simulink model "Z_3Dctrl"  (R2023a)
settings: Solver=ode1  StartTime=0.0  StopTime=inf  FixedStep=0.001  RelTol=1e-3  EnableMultiTasking=on
PostLoadFcn:
  | , if any(exist('dsrtsu_mdlpostloadfcn', 'file') ~= 0), dsrtsu_mdlpostloadfcn('Execute', bdroot); end,
InitFcn:
  | , if any(exist('rtifpga_mdlclblib', 'file') ~= 0), rtifpga_mdlclblib('Init', bdroot); end,
  | [b,a] = butter(6,0.6)
  | z0_default = 0.080001
  | fatness_default = 1
  | offset_default = 0
  | scale_default = 0
  | tic
model workspace (MAT data in the model file):
  Iters = 5
  N_coils = 6
  fatness_default = 1
  running = 0
  z0_default = 0.080001
undefined symbols (not defined in the file or in its folder): a, b, DiscIntNeverNeededParam
libraries: dspstat3 x7, simulink x5, commfilt2 x3, rti2004lib x3, rtilibm x1
(part 1 of 3)
settings Model: DSRTSU_INTERNAL_RTI_VER=620  DSRTSU_INTERNAL_RTI_TYPE=rti1006  DSRTSU_INTERNAL_RTIFPGA=200  DSRTSU_INTERNAL_RTISTBM_VER=23.1  Creator=Administrator  LastModifiedBy=inst
settings SolverCC: AlgebraicLoopSolver=TrustRegion
settings DataIOCC: LimitDataPoints=on  SaveFormat=Array  SignalLoggingSaveFormat=ModelDataLogs  ReturnWorkspaceOutputs=off
settings OptimizationCC: BlockReduction=off  OptimizeBlockIOStorage=off  BufferReuse=off  ReuseModelBlockBuffer=off  ExpressionFolding=off  ExpressionDepthLimit=2147483647  LocalBlockOutputs=off  LifeSpan=inf
settings DebuggingCC: UnderspecifiedInitializationDetection=Classic  MergeDetectMultiDrivingBlocksExec=none  SolverPrmCheckMsg=warning  FcnCallInpInsideContextMsg=warning  UnconnectedInputMsg=warning  UnconnectedOutputMsg=warning  UnconnectedLineMsg=warning  StateNameClashWarn=warning  SFUnexpectedBacktrackingDiag=warning  SFNoUnconditionalDefaultTransitionDiag=warning  SFExecutionAtInitializationDiag=none  ArithmeticOperatorsInVariantConditions=warning
settings HardwareCC: ProdBitPerPointer=32  ProdBitPerSizeT=32  ProdBitPerPtrDiffT=32  ProdLargestAtomicInteger=Integer  ProdWordSize=32  ProdHWDeviceType=Custom Processor->Custom  TargetIntDivRoundTo=Zero  TargetEndianess=LittleEndian  TargetHWDeviceType=Custom Processor->Custom
settings ModelReferenceCC: EnableRefExpFcnMdlSchedulingChecks=on  PropagateSignalLabelsOutOfModel=off
settings SFSimCC: SimUseLocalCustomCode=off  MATLABDynamicMemAlloc=off  CustomCodeUndefinedFunction=UseInterfaceOnly
settings RTWCC: Description=dSPACE DS1006 Hardware Platform  SystemTargetFile=rti1006.tlc  MakeCommand=make_rti  TemplateMakefile=rti1006.tmf  RTWUseLocalCustomCode=off
settings CodeAppCC: StateflowObjectComments=on
settings STFCustomTargetCC: TargetLangStandard=C89/C90 (ANSI)  ParMdlRefBuildCompliant=on  ConcurrentExecutionCompliant=off  GRTInterface=off  UseToolchainInfoCompliant=off  SystemTargetFile=rti1006.tlc
settings GRTTargetCC: TargetLangStandard=C89/C90 (ANSI)  CompOptLevelCompliant=off  ConcurrentExecutionCompliant=off  CombineOutputUpdateFcns=off  MatFileLogging=off  CPPClassGenCompliant=off  UseToolchainInfoCompliant=off  ExtModeMexFile=noextcomm
settings ConfigComp: CovMetricSettings=dw  CovSaveCumulativeToWorkspaceVar=on  CovSaveSingleToWorkspaceVar=on

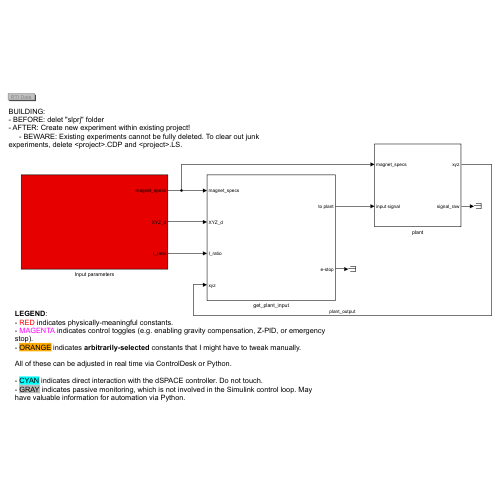
[thumbnail: Simulink's stored preview of the top-level diagram]
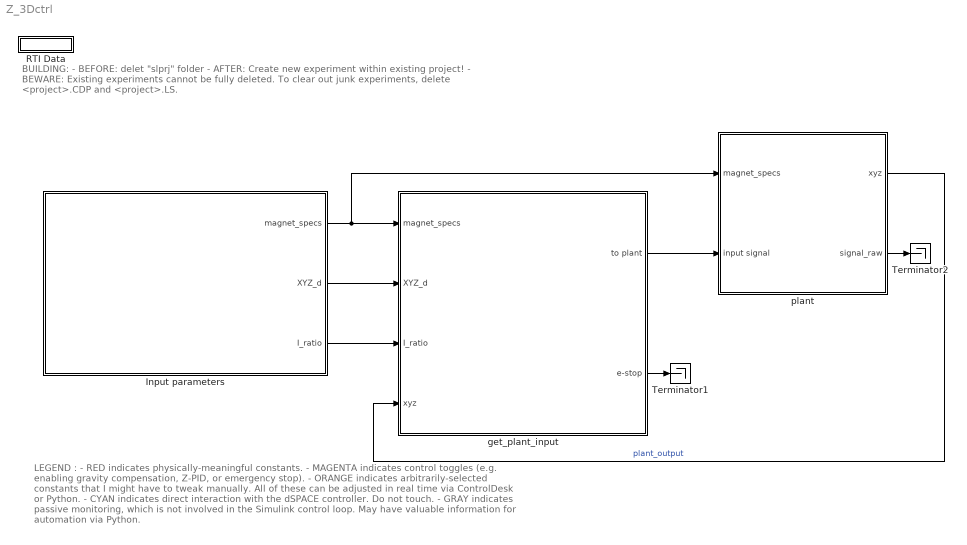
== system Z_3Dctrl ==
  note: BUILDING:
      | - BEFORE: delet "slprj" folder
      | - AFTER: Create new experiment within existing project!
      | - BEWARE: Existing experiments cannot be fully deleted. To clear out junk experiments, delete <project>.CDP and <project>.LS.
  note: LEGEND :
      | - RED indicates physically-meaningful constants.
      | - MAGENTA indicates control toggles (e.g. enabling gravity compensation, Z-PID, or emergency stop).
      | - ORANGE indicates arbitrarily-selected constants that I might have to tweak manually.
      |
      | All of these can be adjusted in real time via ControlDesk or Python.
      |
      | - CYAN indicates direct interaction with the dSPACE controller. Do not touch.
      | - GRAY indicates passive monitoring, which is not involved in the Simulink control loop. May have valuable information for automation via Python.
  Input parameters : Subsystem
  RTI Data : Subsystem  Tag=struct('RTIDataServer',struct('RTIDataServerVs','2','RTIModelDescription','struct(''main'',''Z_1Dctrl_simplified'',''sub'','''',''isMp'',0)'))  LoadFcn="if exist('rtidc'), try,  rtidc('DataHostBlockClbLoad', gcbh); catch, disp(['Warning: ''LoadFcn'' for RTI Data block failed: ' lasterr]); end, end,"  mask(RTI_DATA_HOST){}
      mask help:
      | RTI Data Block.
      | This block is used by RTI to store internal model-dependent data.
      | Please keep this block on the root level of the model. Deleting this block will result in data loss.
      |
      | NEVER DELETE OR COPY THIS BLOCK!
      settings: CopyFcn="if exist('rtidc'), try,  rtidc('DataHostBlockClbCopy', gcbh); catch, disp(['Warning: ''CopyFcn'' for RTI Data block failed: ' lasterr]); end, end,"  DeleteFcn="if exist('rtidc'), try,  rtidc('DataHostBlockClbDelete', gcbh); catch, disp(['Warning: ''DeleteFcn'' for RTI Data block failed: ' lasterr]); end, end,"  ModelCloseFcn="if exist('rtidc'), try,  rtidc('DataHostBlockClbModelClose', gcbh); catch, disp(['Warning: ''ModelCloseFcn'' for RTI Data block failed: ' lasterr]); end, end,"  PreSaveFcn="if exist('rtidc'), try,  rtidc('DataHostBlockClbPreSave', gcbh); catch, disp(['Warning: ''PreSaveFcn'' for RTI Data block failed: ' lasterr]); end, end,"  PostSaveFcn="if exist('rtidc'), try,  rtidc('DataHostBlockClbPostSave', gcbh); catch, disp(['Warning: ''PostSaveFcn'' for RTI Data block failed: ' lasterr]); end, end,"  NameChangeFcn="if exist('rtidc'), try,  rtidc('DataHostBlockClbNameChange', gcbh); catch, disp(['Warning: ''NameChangeFcn'' for RTI Data block failed: ' lasterr]); end, end,"
      mask Help:
      | RTI Data Block.
      | This block is used by RTI to store internal model-dependent data.
      | Please keep this block on the root level of the model. Deleting this block will result in data loss.
      | 
      | NEVER DELETE OR COPY THIS BLOCK!
      mask Display:
      | text(0.5, 0.5, 'RTI Data', 'HorizontalAlignment', 'center');
      | plot([1 0]);
  Terminator1 : Terminator
  Terminator2 : Terminator
  get_plant_input : Subsystem
  plant : Subsystem
  wires:
  Input parameters/1(magnet_specs) -> plant/1(magnet_specs), get_plant_input/1(magnet_specs)
  Input parameters/2(XYZ_d) -> get_plant_input/2(XYZ_d)
  plant/1(xyz) -> get_plant_input/4(xyz)  "plant_output"
  Input parameters/3(I_ratio) -> get_plant_input/3(I_ratio)
  get_plant_input/1(to plant) -> plant/2(input signal)
  get_plant_input/2(e-stop) -> Terminator1/1
  plant/2(signal_raw) -> Terminator2/1

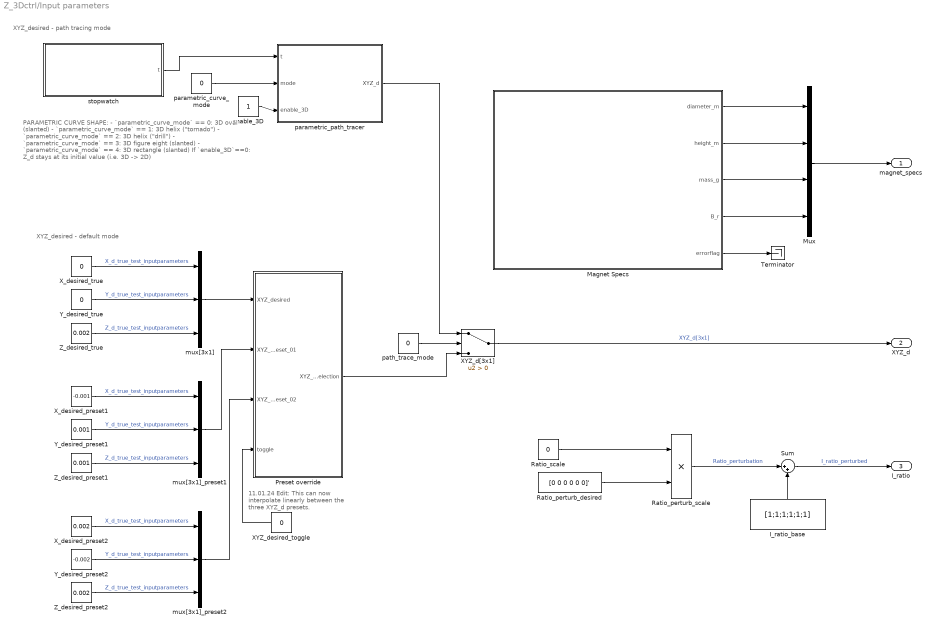
== system Z_3Dctrl/Input parameters ==
  note: XYZ_desired - path tracing mode
  note: PARAMETRIC CURVE SHAPE:
      | - `parametric_curve_mode` == 0: 3D oval (slanted)
      | - `parametric_curve_mode` == 1: 3D helix ("tornado")
      | - `parametric_curve_mode` == 2: 3D helix ("drill")
      | - `parametric_curve_mode` == 3: 3D figure eight (slanted)
      | - `parametric_curve_mode` == 4: 3D rectangle (slanted)
      |
      | If `enable_3D`==0: Z_d stays at its initial value (i.e. 3D -> 2D)
  note: XYZ_desired - default mode
  note: 11.01.24 Edit:
      | This can now interpolate linearly between the three XYZ_d presets.
  I_ratio_base : Constant  Value=[1;1;1;1;1;1]
  Magnet Specs : Subsystem
  Mux : Mux
  Preset override : MATLAB Function  TreatAsAtomicUnit=on
  Ratio_perturb_desired : Constant  Value=[0 0 0 0 0 0]'
  Ratio_perturb_scale : Product
  Ratio_scale : Constant  Value=0
  Sum : Sum  Inputs=|++
  Terminator : Terminator
  XYZ_d[3x1] : Switch  Criteria=u2 > Threshold  SaturateOnIntegerOverflow=off  InputSameDT=off
  XYZ_desired_toggle : Constant  Value=0
  X_desired_preset1 : Constant  Value=-0.001
  X_desired_preset2 : Constant  Value=0.002
  X_desired_true : Constant  Value=0
  Y_desired_preset1 : Constant  Value=0.001
  Y_desired_preset2 : Constant  Value=-0.002
  Y_desired_true : Constant  Value=0
  Z_desired_preset1 : Constant  Value=0.001
  Z_desired_preset2 : Constant  Value=0.002
  Z_desired_true : Constant  Value=0.002
  enable_3D : Constant
  mux[3x1] : Mux  Inputs=3
  mux[3x1]_preset1 : Mux  Inputs=3
  mux[3x1]_preset2 : Mux  Inputs=3
  parametric_curve_mode : Constant  Value=0
  parametric_path_tracer : MATLAB Function  TreatAsAtomicUnit=on
  path_trace_mode : Constant  Value=0
  stopwatch : Subsystem
  magnet_specs : Outport
  XYZ_d : Outport  Port=2
  I_ratio : Outport  Port=3
  wires:
  Magnet Specs/1(diameter_m) -> Mux/1
  Magnet Specs/2(height_m) -> Mux/2
  Magnet Specs/3(mass_g) -> Mux/3
  Magnet Specs/4(B_r) -> Mux/4
  Mux/1 -> magnet_specs/1
  Magnet Specs/5(errorflag) -> Terminator/1
  Z_desired_true/1 -> mux[3x1]/3  "Z_d_true_test_inputparameters"
  Ratio_scale/1 -> Ratio_perturb_scale/1
  Ratio_perturb_desired/1 -> Ratio_perturb_scale/2
  Sum/1 -> I_ratio/1  "I_ratio_perturbed"
  I_ratio_base/1 -> Sum/2
  Ratio_perturb_scale/1 -> Sum/1  "Ratio_perturbation"
  Y_desired_true/1 -> mux[3x1]/2  "Y_d_true_test_inputparameters"
  X_desired_true/1 -> mux[3x1]/1  "X_d_true_test_inputparameters"
  mux[3x1]/1 -> Preset override/1(XYZ_desired)
  Preset override/1(XYZ_desired_selection) -> XYZ_d[3x1]/3
  X_desired_preset1/1 -> mux[3x1]_preset1/1  "X_d_true_test_inputparameters"
  Y_desired_preset1/1 -> mux[3x1]_preset1/2  "Y_d_true_test_inputparameters"
  mux[3x1]_preset1/1 -> Preset override/2(XYZ_preset_01)
  Z_desired_preset1/1 -> mux[3x1]_preset1/3  "Z_d_true_test_inputparameters"
  mux[3x1]_preset2/1 -> Preset override/3(XYZ_preset_02)
  Y_desired_preset2/1 -> mux[3x1]_preset2/2  "Y_d_true_test_inputparameters"
  X_desired_preset2/1 -> mux[3x1]_preset2/1  "X_d_true_test_inputparameters"
  Z_desired_preset2/1 -> mux[3x1]_preset2/3  "Z_d_true_test_inputparameters"
  XYZ_desired_toggle/1 -> Preset override/4(toggle)
  XYZ_d[3x1]/1 -> XYZ_d/1  "XYZ_d[3x1]"
  path_trace_mode/1 -> XYZ_d[3x1]/2
  stopwatch/1(t) -> parametric_path_tracer/1(t)
  parametric_curve_mode/1 -> parametric_path_tracer/2(mode)
  enable_3D/1 -> parametric_path_tracer/3(enable_3D)
  parametric_path_tracer/1(XYZ_d) -> XYZ_d[3x1]/1

== system Z_3Dctrl/RTI Data ==
  RTI Data Store : Subsystem  Tag="struct('private',struct('version',struct('dsVer',uint32(2),'dsVerCreation',uint32(2),'RTI',struct('ver','6.2','type','RTI1006')),'access',struct('type','Model','isPerm',1,'created',['29-Jul-2010 10:53:51'],'modified',['20-Nov-2024 19:16:55'],'location','')),'public',struct('main',struct('data',[]),'sub',struct('name',{{'Z_1Dctrl_simplified'}},'data',{{struct('TH',struct('thTaskInfo',struct('taskType',{'TIMER','HWINT','TMRINT','SWINT','GLINT'},'tasksNumOf',{1,0,0,0,0},'srcIds',{{'TIMERA'},{},{},{},{}},'taskNames',{{['Timer Task 1']},{},{},{},{}})),'th_tc',struct('dataType','TASK','taskGroupId','','taskGroupList',{{}},'taskSchedulingPolicy','FCFS','taskType','TIMER','blkh',-1,'srcId','TIMERA','srcSgnName',['Timer A interrupt'],'srcCpuName','','taskName',['Timer Task 1  [0.001] s'],'taskNameDisplayExt','','smplTime',0.001,'smplTimeOffs',0,'hasFixedPriority',0,'priority',1,'hasFixedOvc',0,'ovcType',1,'ovcMax',1),'tc_th',struct('dataType','TASK','taskGroupId','','taskGroupList',{{}},'taskSchedulingPolicy','FCFS','taskType','TIMER','blkh',-1,'srcId','TIMERA','srcSgnName',['Timer A interrupt'],'srcCpuName','','taskName',['Timer Task 1  [0.001] s'],'taskNameDisplayExt','','smplTime',0.001,'smplTimeOffs',0,'hasFixedPriority',0,'priority',1,'hasFixedOvc',0,'ovcType',1,'ovcMax',1))}})))"  mask(RTI_DATA_STORE){}
      mask help:
      | RTI Data Store Block. This block is used by RTI to store internal model dependent data. Deleting this block will result in data loss.
      |
      | NEVER DELETE, COPY, OR MODIFY THIS BLOCK!
      mask Help:
      | RTI Data Store Block. This block is used by RTI to store internal model dependent data. Deleting this block will result in data loss.
      | 
      | NEVER DELETE, COPY, OR MODIFY THIS BLOCK!
      mask Display: text(0.5, 0.5, ' ', 'HorizontalAlignment', 'center');

== system Z_3Dctrl/get_plant_input ==
  note: Inputs
  magnet_specs : Inport
  XYZ_d : Inport  Port=2
  I_ratio : Inport  Port=3
  xyz : Inport  Port=4
  Z_1dctrl : Subsystem
  to plant : Outport
  e-stop : Outport  Port=2
  wires:
  XYZ_d/1 -> Z_1dctrl/4(XYZd)
  xyz/1 -> Z_1dctrl/3(xyz)
  Z_1dctrl/1(to plant) -> to plant/1
  magnet_specs/1 -> Z_1dctrl/1(magnet specs)
  I_ratio/1 -> Z_1dctrl/2(I_ratio)
  Z_1dctrl/2(e-stop) -> e-stop/1

== system Z_3Dctrl/plant ==
  note: NOTE:
      | Output signal contains:
      | - x_pos : Centered, smoothed "x" [m] (not used in control yet)
      | - y_pos : Centered, smoothed "y" [m] (not used in control yet)
      | - z_pos : Centered, smoothed "z" [m] (to be used in derivative-related calculations ONLY)
      | - z_pos_raw : Centered but otherwise unprocessed "z" [m] (to be used in "PI" ONLY)
  magnet_specs : Inport  PortDimensions=[1 4]
  input signal : Inport  Port=2
  DS2103_B1 : rtilibm/DS2103/DS2103_B1  BoardNo=1  ChannelNos=[1 2 4 6 8 9 10 11 12 18 19 20]  Range=[10 10 10 10 10 10 10 10 10 10 10 10 10 10 10 10 10 10 10 10 10 10 10 10 10 10 10 10 10 10 10 10]  IOErrorMode=[1 1 1 1 1 1 1 1]  InitValue=[0 0 0 0 0 0 0 0 0 0 0 0 0 0 0 0 0 0 0 0 0 0 0 0 0 0 0 0 0 0 0 0]  TermMode=[0 0 0 0 0 0 0 1 1 1 1 1 1 1 1 1 1 1 1 1 1 1 1 1 1 1 1 1 1 1 1 1]  TermValue=[0 0 0 0 0 0 0 0 0 0 0 0 0 0 0 0 0 0 0 0 0 0 0 0 0 0 0 0 0 0 0 0]  DialogFcn=gui2103  UnitName={ 'DS2103_B' }  UnitValues={ 1 }  DSProperties=struct('RTI',struct('Version',uint32(1),'BlockType',struct('isSLSource',uint8(0),'isSLSink',uint8(1),'isHWSource',uint8(0),'isHWSink',uint8(1),'isSetup',uint8(0),'isInline',uint8(1),'isNonInline',uint8(0),'isInterrupt',uint8(0),'isChannelwise',uint8(0)),'IOBoardType','DS2103','UnitType','DAC','Identifier','DACMUX','DialogType','ML','BlockSet','NONE','SlaveProcessor','NONE'))
      settings: SourceProductName=dSPACE RTI1006
  Demux : Demux
  Mux : Mux  Inputs=3
  Position Determination1 : Subsystem  TreatAsAtomicUnit=on
  Terminator : Terminator
  Terminator2 : Terminator
  output signal : Subsystem
  xyz : Outport
  signal_raw : Outport  Port=2
  wires:
  input signal/1 -> DS2103_B1/1
  Demux/4 -> Terminator/1  "B_r"
  Demux/1 -> Position Determination1/1(height_m)  "diameter_m"
  Demux/2 -> Position Determination1/2(diameter_m)  "height_m"
  Demux/3 -> Terminator2/1  "mass_g"
  Position Determination1/1(x_SAR(m)) -> Mux/1  "x_SAR"
  Position Determination1/2(y_SAR(m)) -> Mux/2  "y_SAR"
  Position Determination1/3(z_SAR(m)) -> Mux/3  "z_SAR"
  output signal/1(plant signals) -> signal_raw/1, Position Determination1/3(plant signals)
  Mux/1 -> xyz/1
  magnet_specs/1 -> Demux/1

== system Z_3Dctrl/Input parameters/Magnet Specs ==
  note: NOTE: Xiaodong lists the magnet as having 10mm height and 10mm diameter. However, height is closer to 11-12mm. Diameter is closer to ????.
  Diameter : Constant  Value=0.635
  Height : Constant  Value=0.635
  Magnet Physical Specs : MATLAB Function  TreatAsAtomicUnit=on
  Mass (g) : Constant  Value=1.5081
  Units : StringConstant  Commented=on  String="\"cm\""
  Units_mode : Constant  Value=2
  mag-field Br value (in T or G) : Constant  Value=1.45
  string to unit mode : Subsystem  Commented=on
  diameter_m : Outport
  height_m : Outport  Port=2
  mass_g : Outport  Port=3
  B_r : Outport  Port=4
  errorflag : Outport  Port=5
  wires:
  Diameter/1 -> Magnet Physical Specs/2(diameter)
  Height/1 -> Magnet Physical Specs/3(height)
  Mass (g)/1 -> Magnet Physical Specs/4(mass)
  Magnet Physical Specs/1(diameter_m) -> diameter_m/1
  Magnet Physical Specs/2(height_m) -> height_m/1
  Magnet Physical Specs/4(B_r) -> B_r/1
  Magnet Physical Specs/3(mass_g) -> mass_g/1
  Magnet Physical Specs/5(errorflag) -> errorflag/1
  Units_mode/1 -> Magnet Physical Specs/1(unit_mode)  "unit_mode"
  mag-field Br value (in T or G)/1 -> Magnet Physical Specs/5(magnet_remanence_t)
  Units/1 -> string to unit mode/1(In1)

== system Z_3Dctrl/Input parameters/stopwatch ==
  note: INSTRUCTIONS:
      | - `play_or_pause` == 1: PLAY (i.e. stopwatch accumulates by `speedmult` per second)
      | - `play_or_pause` == 0: PAUSE (i.e. stopwatch freezes)
      | - `reset` increases : RESET (i.e. stopwatch resets back to 0, without affecting PLAY or PAUSE
  ms_to_s : Gain
  play_or_pause : Constant  Value=0
  reset : Constant  Value=0
  speedmult : Gain
  stopwatch : DiscreteIntegrator  ExternalReset=rising  SampleTime=-1  ICPrevOutput=DiscIntNeverNeededParam  ICPrevScaledInput=DiscIntNeverNeededParam
  t : Outport
  wires:
  ms_to_s/1 -> speedmult/1
  play_or_pause/1 -> ms_to_s/1
  reset/1 -> stopwatch/2
  speedmult/1 -> stopwatch/1
  stopwatch/1 -> t/1

== system Z_3Dctrl/RTI Data/RTI Data Store ==
  RTI Data Store : Subsystem  mask(RTI_DATA_STORE){}
      mask help:
      | RTI Data Store Block. This block is used by RTI to store internal model dependent data. Deleting this block will result in data loss.
      |
      | NEVER DELETE, COPY, OR MODIFY THIS BLOCK!
      mask Help:
      | RTI Data Store Block. This block is used by RTI to store internal model dependent data. Deleting this block will result in data loss.
      | 
      | NEVER DELETE, COPY, OR MODIFY THIS BLOCK!
      mask Display: text(0.5, 0.5, ' ', 'HorizontalAlignment', 'center');

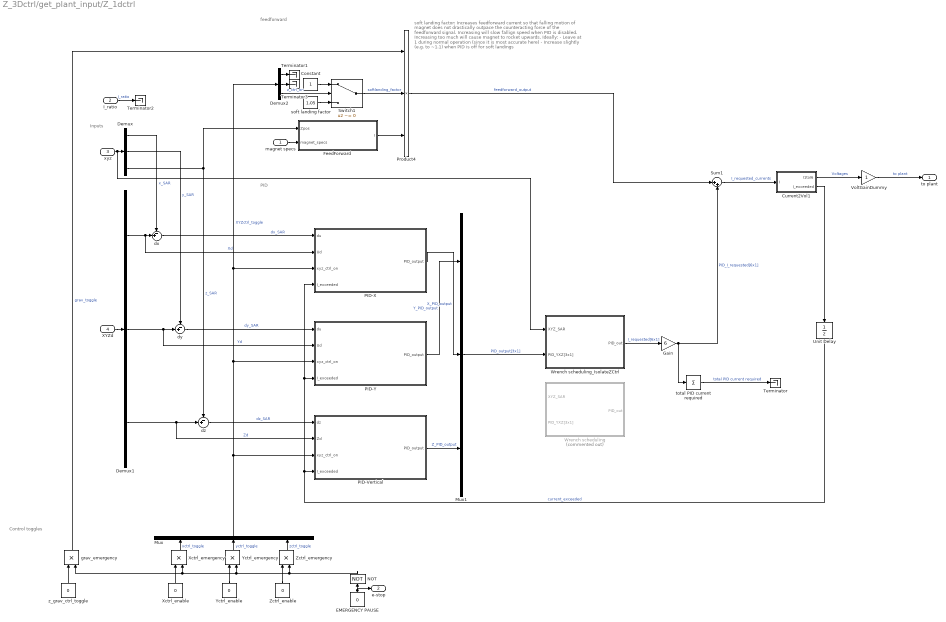
== system Z_3Dctrl/get_plant_input/Z_1dctrl ==
  note: feedforward
  note: Inputs
  note: soft landing factor:
      | Increases feedforward current so that falling motion of magnet does not drastically outpace the counteracting force of the feedforward signal.
      | Increasing will slow fallign speed when PID is disabled. Increasing too much will cause magnet to rocket upwards.
      |
      | Ideally:
      | - Leave at 1 during normal operation (since it is most accurate here)
      | - Increase slightly (e.g. to ~1.1) when PID is off for soft landings
  note: PID
  note: Control toggles
  magnet specs : Inport
  I_ratio : Inport  Port=2
  xyz : Inport  Port=3
  XYZd : Inport  Port=4
  Constant : Constant
  Current2Vol1 : Subsystem  TreatAsAtomicUnit=on
  Demux : Demux  Outputs=3
  Demux1 : Demux  Outputs=3
  Demux2 : Demux  Outputs=3
  EMERGENCY PAUSE : Constant  Value=0
  FeedForward : Subsystem  TreatAsAtomicUnit=on
  Gain : Gain  Gain=6
  Mux : Mux  Inputs=3
  Mux1 : Mux  Inputs=3
  NOT : Logic  Operator=NOT  IconShape=distinctive  AllPortsSameDT=off  OutDataTypeStr=boolean
  PID-Vertical : Subsystem  TreatAsAtomicUnit=on
  PID-X : Subsystem  TreatAsAtomicUnit=on
  PID-Y : Subsystem  TreatAsAtomicUnit=on
  Product4 : Product  Inputs=3
  Sum1 : Sum  Inputs=|++
  Switch1 : Switch  Criteria=u2 ~= 0  Threshold=1  SaturateOnIntegerOverflow=off  InputSameDT=off
  Terminator{,1..3} (4 alike) : Terminator
  Unit Delay : UnitDelay  InitialCondition=1  SampleTime=-1  HasFrameUpgradeWarning=on
  VoltGainDummy : Gain
  Wrench scheduling : Subsystem  Commented=on
  Wrench scheduling_IsolateZCtrl : Subsystem
  Xctrl_emergency : Product
  Xctrl_enable : Constant  Value=0
  Yctrl_emergency : Product
  Yctrl_enable : Constant  Value=0
  Zctrl_emergency : Product
  Zctrl_enable : Constant  Value=0
  dx : Sum  Inputs=-+|
  dy : Sum  Inputs=-+|
  dz : Sum  Inputs=-+|
  grav_emergency : Product
  soft landing factor : Constant  Value=1.05
  total PID current required : Sum  Inputs=+
  z_grav_ctrl_toggle : Constant  Value=0
  to plant : Outport
  e-stop : Outport  Port=2
  wires:
  Sum1/1 -> Current2Vol1/1(I)  "I_requested_currents"
  Unit Delay/1 -> PID-Vertical/4(I_exceeded), PID-X/4(I_exceeded), PID-Y/4(I_exceeded)  "current_exceeded"
  z_grav_ctrl_toggle/1 -> grav_emergency/1
  Zctrl_enable/1 -> Zctrl_emergency/1
  Mux/1 -> PID-Vertical/3(xyz_ctrl_on), PID-Y/3(xyz_ctrl_on), Demux2/1, PID-X/3(xyz_ctrl_on)  "XYZctrl_toggle"
  grav_emergency/1 -> Product4/1  "grav_toggle"
  VoltGainDummy/1 -> to plant/1  "to plant"
  Current2Vol1/1(I1toI6) -> VoltGainDummy/1  "Voltages"
  Current2Vol1/2(I_exceeded) -> Unit Delay/1
  EMERGENCY PAUSE/1 -> e-stop/1, NOT/1
  PID-Vertical/1(PID_output) -> Mux1/3  "Z_PID_output"
  FeedForward/1(I) -> Product4/3
  magnet specs/1 -> FeedForward/2(magnet_specs)
  Demux1/3 -> dz/2, PID-Vertical/2(Zd)  "Zd"
  dz/1 -> PID-Vertical/1(dz)  "dz_SAR"
  Constant/1 -> Switch1/1
  soft landing factor/1 -> Switch1/3
  Switch1/1 -> Product4/2  "softlanding_factor"
  Demux/3 -> FeedForward/1(Zpos), dz/1  "z_SAR"
  Demux/1 -> dx/1  "x_SAR"
  Demux/2 -> dy/1  "y_SAR"
  xyz/1 -> Wrench scheduling_IsolateZCtrl/1(XYZ_SAR), Demux/1
  Product4/1 -> Sum1/1  "feedforward_output"
  I_ratio/1 -> Terminator2/1  "I_ratio"
  XYZd/1 -> Demux1/1
  Demux1/2 -> PID-Y/2(Ud), dy/2  "Yd"
  Demux1/1 -> PID-X/2(Ud), dx/2  "Xd"
  dy/1 -> PID-Y/1(du)  "dy_SAR"
  dx/1 -> PID-X/1(du)  "dx_SAR"
  Xctrl_enable/1 -> Xctrl_emergency/1
  NOT/1 -> Yctrl_emergency/2, Xctrl_emergency/2, grav_emergency/2, Zctrl_emergency/2
  Yctrl_enable/1 -> Yctrl_emergency/1
  Xctrl_emergency/1 -> Mux/1  "xctrl_toggle"
  Yctrl_emergency/1 -> Mux/2  "yctrl_toggle"
  Zctrl_emergency/1 -> Mux/3  "zctrl_toggle"
  PID-Y/1(PID_output) -> Mux1/1  "Y_PID_output"
  PID-X/1(PID_output) -> Mux1/2  "X_PID_output"
  Mux1/1 -> Wrench scheduling_IsolateZCtrl/2(PID_YXZ[3x1])  "PID_output[3x1]"
  Gain/1 -> total PID current required/1, Sum1/2  "PID_I_requested[6x1]"
  Wrench scheduling_IsolateZCtrl/1(PID_out) -> Gain/1  "I_requested[6x1]"
  Demux2/2 -> Terminator3/1
  Demux2/1 -> Terminator1/1
  Demux2/3 -> Switch1/2  "z_ctrl_on"
  total PID current required/1 -> Terminator/1  "total PID current required"

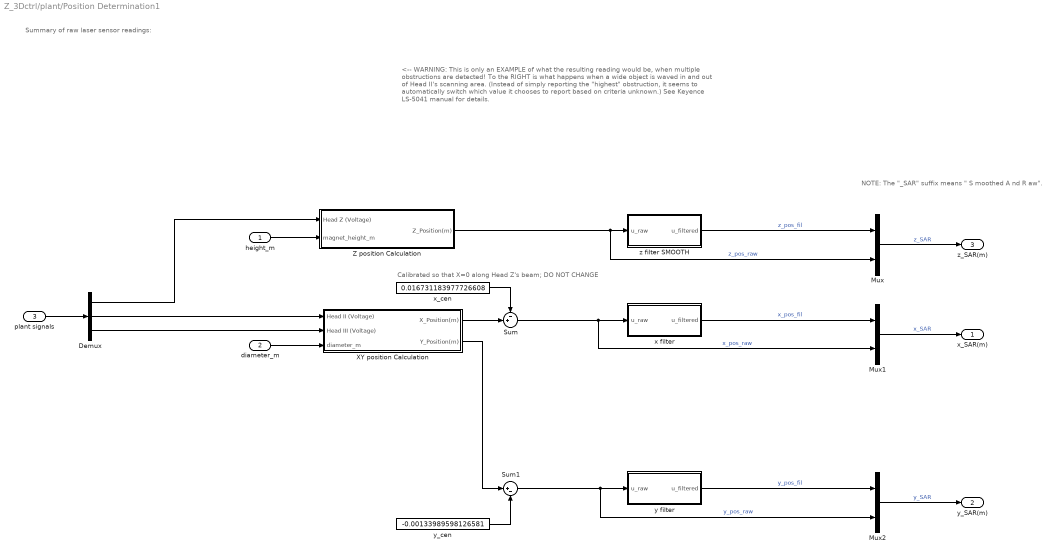
== system Z_3Dctrl/plant/Position Determination1 ==
  note: NOTE:
      | The "_SAR" suffix means " S moothed A nd R aw".
  note: <-- WARNING:
      | This is only an EXAMPLE of what the resulting reading would be, when multiple obstructions are detected!
      | To the RIGHT is what happens when a wide object is waved in and out of Head II's scanning area. (Instead of simply reporting the "highest" obstruction, it seems to automatically switch which value it chooses to report based on criteria unknown.)
      | See Keyence LS-5041 manual for details.
  note: Calibrated so that X=0 along Head Z's beam; DO NOT CHANGE
  note: Summary of raw laser sensor readings:
  height_m : Inport
  diameter_m : Inport  Port=2
  plant signals : Inport  Port=3
  Demux : Demux  Outputs=3
  Mux : Mux  Inputs=2
  Mux1 : Mux  Inputs=2
  Mux2 : Mux  Inputs=2
  Sum : Sum  Inputs=-+|
  Sum1 : Sum  Inputs=|+-
  XY position Calculation : Subsystem
  Z position Calculation : Subsystem
  x filter : Subsystem
  x_cen : Constant  Value=0.016731183977726608
  y filter : Subsystem
  y_cen : Constant  Value=-0.00133989598126581
  z filter SMOOTH : Subsystem
  x_SAR(m) : Outport
  y_SAR(m) : Outport  Port=2
  z_SAR(m) : Outport  Port=3
  wires:
  XY position Calculation/2(Y_Position(m)) -> Sum1/1
  XY position Calculation/1(X_Position(m)) -> Sum/2
  Z position Calculation/1(Z_Position(m)) -> Mux/2, z filter SMOOTH/1(u_raw)  "z_pos_raw"
  x_cen/1 -> Sum/1
  y_cen/1 -> Sum1/2
  Sum/1 -> Mux1/2, x filter/1(u_raw)  "x_pos_raw"
  Sum1/1 -> Mux2/2, y filter/1(u_raw)  "y_pos_raw"
  height_m/1 -> Z position Calculation/2(magnet_height_m)
  diameter_m/1 -> XY position Calculation/3(diameter_m)
  Demux/1 -> Z position Calculation/1(Head Z (Voltage))
  Demux/2 -> XY position Calculation/1(Head II (Voltage))
  Demux/3 -> XY position Calculation/2(Head III (Voltage))
  z filter SMOOTH/1(u_filtered) -> Mux/1  "z_pos_fil"
  x filter/1(u_filtered) -> Mux1/1  "x_pos_fil"
  y filter/1(u_filtered) -> Mux2/1  "y_pos_fil"
  plant signals/1 -> Demux/1
  Mux/1 -> z_SAR(m)/1  "z_SAR"
  Mux1/1 -> x_SAR(m)/1  "x_SAR"
  Mux2/1 -> y_SAR(m)/1  "y_SAR"

== system Z_3Dctrl/plant/output signal ==
  DS2004ADC_BL1 : rti2004lib/DS2004ADC_BL1  DSProperties=struct('RTI',struct('Version',uint32(1),'BlockType',struct('isSLSource',uint8(1),'isSLSink',uint8(1),'isHWSource',uint8(0),'isHWSink',uint8(1),'isSetup',uint8(0),'isInline',uint8(1),'isNonInline',uint8(0),'isInterrupt',uint8(0),'isChannelwise',uint8(1)),'IOBoardType','DS2004','UnitType','ADC','Identifier','ADC','DialogType','ML','BlockSet','NONE','SlaveProcessor','NONE'))  RTIBlockInterface=struct('InputPortsActive',0,'InputPortsWidth',int32(1),'InputPortsDataType',{{'SS_BOOLEAN'}},'InputPortsName',{{'Continue'}},'OutputPortsActive',[1 0],'OutputPortsWidth',int32([1 1]),'OutputPortsDataType',{{'SS_DOUBLE','SS_UINT8'}},'OutputPortsName',{{'ADC','Status'}},'DialogFcn','rti2004adcgui','SampleTime',{{-1}},'InitLevel',3,'IconTransparency','on','BlockDisplay',{{['DS2004 ADC\nBoard: 1\nChannel: 1'],'center'}},'BlockName',struct('Token',{{'DS2004ADC_BL1'}}))  RTIBlockParameters=struct('ADCSWStartDisable',{{0,'OFF',[0 1]}},'BoardNo',{{1,'OFF',[1 16]}},'ChannelNo',{{1,'OFF',[1 16]}},'ConversionMode',{{1,'OFF',[1 2]}},'SampleMode',{{1,'OFF',[1 2]}},'TriggerSource',{{1,'OFF',[1 5]}},'EdgePolarity',{{1,'OFF',[1 2]}},'ConversionTriggerSource',{{2,'OFF',[1 6]}},'ConversionEdgePolarity',{{1,'OFF',[1 2]}},'ConversionPeriod',{{1e-6,'OFF',[]}},'ConversionPeriodCheck',{{0,'OFF',[]}},'BurstTriggerSource',{{1,'OFF',[1 6]}},'BurstEdgePolarity',{{1,'OFF',[1 2]}},'BurstSize',{{10,'OFF',[]}},'BurstSizeCheck',{{0,'OFF',[]}},'DataSetOffset',{{0,'OFF',[]}},'DataSetOffsetCheck',{{0,'OFF',[]}},'DataSetLength',{{1,'OFF',[]}},'DataSetLengthCheck',{{0,'OFF',[]}},'ReadMode',{{1,'OFF',[1 2]}},'SampleTime',{{-1,'OFF',[-1 inf]}},'SampleTimeCheck',{{1,'OFF',[]}},'InputVoltageRange',{{2,'OFF',[1 2]}},'StatusPortEnable',{{0,'OFF',[0 1]}},'TLCFileName',{{'rti2004adc','OFF',[]}})  RTISFcnParameters=struct('ADCSWStartDisable','int32','BoardNo','int32','ChannelNo','int32','ConversionMode','int32','SampleMode','int32','TriggerSource','int32','EdgePolarity','int32','ConversionTriggerSource','int32','ConversionEdgePolarity','int32','ConversionPeriod','double','BurstTriggerSource','int32','BurstEdgePolarity','int32','BurstSize','int32','DataSetOffset','int32','DataSetLength','int32','ReadMode','int32','SampleTime','double','InputVoltageRange','int32','StatusPortEnable','int32','TLCFileName','char')  RTIBlockParaDefault=struct('ADCSWStartDisable',0,'BoardNo',1,'ChannelNo',1,'ConversionMode',1,'SampleMode',1,'TriggerSource',1,'EdgePolarity',1,'ConversionTriggerSource',2,'ConversionEdgePolarity',1,'ConversionPeriod',1e-6,'ConversionPeriodCheck',0,'BurstTriggerSource',1,'BurstEdgePolarity',1,'BurstSize',10,'BurstSizeCheck',0,'DataSetOffset',0,'DataSetOffsetCheck',0,'DataSetLength',1,'DataSetLengthCheck',0,'ReadMode',1,'SampleTime',-1,'SampleTimeCheck',1,'InputVoltageRange',2,'StatusPortEnable',0,'TLCFileName','rti2004adc')
  DS2004ADC_BL2 : rti2004lib/DS2004ADC_BL1  DSProperties=struct('RTI',struct('Version',uint32(1),'BlockType',struct('isSLSource',uint8(1),'isSLSink',uint8(1),'isHWSource',uint8(0),'isHWSink',uint8(1),'isSetup',uint8(0),'isInline',uint8(1),'isNonInline',uint8(0),'isInterrupt',uint8(0),'isChannelwise',uint8(1)),'IOBoardType','DS2004','UnitType','ADC','Identifier','ADC','DialogType','ML','BlockSet','NONE','SlaveProcessor','NONE'))  RTIBlockInterface=struct('InputPortsActive',0,'InputPortsWidth',int32(1),'InputPortsDataType',{{'SS_BOOLEAN'}},'InputPortsName',{{'Continue'}},'OutputPortsActive',[1 0],'OutputPortsWidth',int32([1 1]),'OutputPortsDataType',{{'SS_DOUBLE','SS_UINT8'}},'OutputPortsName',{{'ADC','Status'}},'DialogFcn','rti2004adcgui','SampleTime',{{-1}},'InitLevel',3,'IconTransparency','on','BlockDisplay',{{['DS2004 ADC\nBoard: 1\nChannel: 2'],'center'}},'BlockName',struct('Token',{{'DS2004ADC_BL1'}}))  RTIBlockParameters=struct('ADCSWStartDisable',{{0,'OFF',[0 1]}},'BoardNo',{{1,'OFF',[1 16]}},'ChannelNo',{{2,'OFF',[1 16]}},'ConversionMode',{{1,'OFF',[1 2]}},'SampleMode',{{1,'OFF',[1 2]}},'TriggerSource',{{1,'OFF',[1 5]}},'EdgePolarity',{{1,'OFF',[1 2]}},'ConversionTriggerSource',{{2,'OFF',[1 6]}},'ConversionEdgePolarity',{{1,'OFF',[1 2]}},'ConversionPeriod',{{'1e-006','OFF',[]}},'ConversionPeriodCheck',{{0,'OFF',[]}},'BurstTriggerSource',{{1,'OFF',[1 6]}},'BurstEdgePolarity',{{1,'OFF',[1 2]}},'BurstSize',{{'10','OFF',[]}},'BurstSizeCheck',{{0,'OFF',[]}},'DataSetOffset',{{'0','OFF',[]}},'DataSetOffsetCheck',{{0,'OFF',[]}},'DataSetLength',{{'1','OFF',[]}},'DataSetLengthCheck',{{0,'OFF',[]}},'ReadMode',{{1,'OFF',[1 2]}},'SampleTime',{{'-1','OFF',[-1 inf]}},'SampleTimeCheck',{{1,'OFF',[]}},'InputVoltageRange',{{2,'OFF',[1 2]}},'StatusPortEnable',{{0,'OFF',[0 1]}},'TLCFileName',{{'rti2004adc','OFF',[]}})  RTISFcnParameters=struct('ADCSWStartDisable','int32','BoardNo','int32','ChannelNo','int32','ConversionMode','int32','SampleMode','int32','TriggerSource','int32','EdgePolarity','int32','ConversionTriggerSource','int32','ConversionEdgePolarity','int32','ConversionPeriod','double','BurstTriggerSource','int32','BurstEdgePolarity','int32','BurstSize','int32','DataSetOffset','int32','DataSetLength','int32','ReadMode','int32','SampleTime','double','InputVoltageRange','int32','StatusPortEnable','int32','TLCFileName','char')  RTIBlockParaDefault=struct('ADCSWStartDisable',0,'BoardNo',1,'ChannelNo',1,'ConversionMode',1,'SampleMode',1,'TriggerSource',1,'EdgePolarity',1,'ConversionTriggerSource',2,'ConversionEdgePolarity',1,'ConversionPeriod',1e-6,'ConversionPeriodCheck',0,'BurstTriggerSource',1,'BurstEdgePolarity',1,'BurstSize',10,'BurstSizeCheck',0,'DataSetOffset',0,'DataSetOffsetCheck',0,'DataSetLength',1,'DataSetLengthCheck',0,'ReadMode',1,'SampleTime',-1,'SampleTimeCheck',1,'InputVoltageRange',2,'StatusPortEnable',0,'TLCFileName','rti2004adc')
  DS2004ADC_BL3 : rti2004lib/DS2004ADC_BL1  DSProperties=struct('RTI',struct('Version',uint32(1),'BlockType',struct('isSLSource',uint8(1),'isSLSink',uint8(1),'isHWSource',uint8(0),'isHWSink',uint8(1),'isSetup',uint8(0),'isInline',uint8(1),'isNonInline',uint8(0),'isInterrupt',uint8(0),'isChannelwise',uint8(1)),'IOBoardType','DS2004','UnitType','ADC','Identifier','ADC','DialogType','ML','BlockSet','NONE','SlaveProcessor','NONE'))  RTIBlockInterface=struct('InputPortsActive',0,'InputPortsWidth',int32(1),'InputPortsDataType',{{'SS_BOOLEAN'}},'InputPortsName',{{'Continue'}},'OutputPortsActive',[1 0],'OutputPortsWidth',int32([1 1]),'OutputPortsDataType',{{'SS_DOUBLE','SS_UINT8'}},'OutputPortsName',{{'ADC','Status'}},'DialogFcn','rti2004adcgui','SampleTime',{{-1}},'InitLevel',3,'IconTransparency','on','BlockDisplay',{{['DS2004 ADC\nBoard: 1\nChannel: 3'],'center'}},'BlockName',struct('Token',{{'DS2004ADC_BL1'}}))  RTIBlockParameters=struct('ADCSWStartDisable',{{0,'OFF',[0 1]}},'BoardNo',{{1,'OFF',[1 16]}},'ChannelNo',{{3,'OFF',[1 16]}},'ConversionMode',{{1,'OFF',[1 2]}},'SampleMode',{{1,'OFF',[1 2]}},'TriggerSource',{{1,'OFF',[1 5]}},'EdgePolarity',{{1,'OFF',[1 2]}},'ConversionTriggerSource',{{2,'OFF',[1 6]}},'ConversionEdgePolarity',{{1,'OFF',[1 2]}},'ConversionPeriod',{{'1e-006','OFF',[]}},'ConversionPeriodCheck',{{0,'OFF',[]}},'BurstTriggerSource',{{1,'OFF',[1 6]}},'BurstEdgePolarity',{{1,'OFF',[1 2]}},'BurstSize',{{'10','OFF',[]}},'BurstSizeCheck',{{0,'OFF',[]}},'DataSetOffset',{{'0','OFF',[]}},'DataSetOffsetCheck',{{0,'OFF',[]}},'DataSetLength',{{'1','OFF',[]}},'DataSetLengthCheck',{{0,'OFF',[]}},'ReadMode',{{1,'OFF',[1 2]}},'SampleTime',{{'-1','OFF',[-1 inf]}},'SampleTimeCheck',{{1,'OFF',[]}},'InputVoltageRange',{{2,'OFF',[1 2]}},'StatusPortEnable',{{0,'OFF',[0 1]}},'TLCFileName',{{'rti2004adc','OFF',[]}})  RTISFcnParameters=struct('ADCSWStartDisable','int32','BoardNo','int32','ChannelNo','int32','ConversionMode','int32','SampleMode','int32','TriggerSource','int32','EdgePolarity','int32','ConversionTriggerSource','int32','ConversionEdgePolarity','int32','ConversionPeriod','double','BurstTriggerSource','int32','BurstEdgePolarity','int32','BurstSize','int32','DataSetOffset','int32','DataSetLength','int32','ReadMode','int32','SampleTime','double','InputVoltageRange','int32','StatusPortEnable','int32','TLCFileName','char')  RTIBlockParaDefault=struct('ADCSWStartDisable',0,'BoardNo',1,'ChannelNo',1,'ConversionMode',1,'SampleMode',1,'TriggerSource',1,'EdgePolarity',1,'ConversionTriggerSource',2,'ConversionEdgePolarity',1,'ConversionPeriod',1e-6,'ConversionPeriodCheck',0,'BurstTriggerSource',1,'BurstEdgePolarity',1,'BurstSize',10,'BurstSizeCheck',0,'DataSetOffset',0,'DataSetOffsetCheck',0,'DataSetLength',1,'DataSetLengthCheck',0,'ReadMode',1,'SampleTime',-1,'SampleTimeCheck',1,'InputVoltageRange',2,'StatusPortEnable',0,'TLCFileName','rti2004adc')
  Head II (V) : Gain  Gain=10
  Head III (V) : Gain  Gain=10
  Head Z (V) : Gain  Gain=10
  Mux : Mux  Inputs=3
  output signal diagnostics : Subsystem
  plant signals : Outport
  wires:
  DS2004ADC_BL1/1 -> Head Z (V)/1
  DS2004ADC_BL2/1 -> Head III (V)/1
  DS2004ADC_BL3/1 -> Head II (V)/1
  Head Z (V)/1 -> Mux/1
  Head II (V)/1 -> Mux/2
  Head III (V)/1 -> Mux/3
  Mux/1 -> output signal diagnostics/1(H123_raw), plant signals/1  "H123_raw"

== system Z_3Dctrl/Input parameters/Magnet Specs/string to unit mode ==
  In1 : Inport
  Gain : Gain
  Gain1 : Gain  Gain=2
  Gain2 : Gain  Gain=3
  Gain3 : Gain  Gain=4
  String Compare{,1..3} (4 alike) : StringCompare
  Sum : Sum  Inputs=|++++|
  cm : StringConstant  String="\"cm\""
  in : StringConstant  String="\"in\""
  m : StringConstant  String="\"m\""
  mm : StringConstant  String="\"mm\""
  unit_mode : Outport
  wires:
  In1/1 -> String Compare3/1, String Compare2/1, String Compare/1, String Compare1/1
  m/1 -> String Compare/2
  cm/1 -> String Compare1/2
  mm/1 -> String Compare2/2
  in/1 -> String Compare3/2
  String Compare/1 -> Gain/1
  String Compare1/1 -> Gain1/1
  String Compare2/1 -> Gain2/1
  String Compare3/1 -> Gain3/1
  Sum/1 -> unit_mode/1
  Gain/1 -> Sum/1
  Gain1/1 -> Sum/2
  Gain2/1 -> Sum/3
  Gain3/1 -> Sum/4

== system Z_3Dctrl/RTI Data/RTI Data Store/RTI Data Store ==
  RTI Data Store : Subsystem  mask(RTI_DATA_STORE){}
      mask help:
      | RTI Data Store Block. This block is used by RTI to store internal model dependent data. Deleting this block will result in data loss.
      |
      | NEVER DELETE, COPY, OR MODIFY THIS BLOCK!
      mask Help:
      | RTI Data Store Block. This block is used by RTI to store internal model dependent data. Deleting this block will result in data loss.
      | 
      | NEVER DELETE, COPY, OR MODIFY THIS BLOCK!
      mask Display: text(0.5, 0.5, ' ', 'HorizontalAlignment', 'center');

== system Z_3Dctrl/get_plant_input/Z_1dctrl/Current2Vol1 ==
  note: Signal 1-2-4-6-5-1-2-3-4-3-5-6
  note: Amplifier takes an input voltage and outputs a current.
      | i = 0.355v , or v = 2.8169014i
      |
      | (where " i " is the desired current flowing through the coils, and " v " is the input voltage required to get this current!)
      |
      | (Notice that the v is multiplied by 0.1 before being sent to the dSPACE controller. Not sure why this is.)
  I : Inport
  Demux1 : Demux  Outputs=6
  Gain2 : Gain  Gain=.1
  Gain4 : Gain  Gain=2.8169014
  Mux2 : Mux  Inputs=6
  Mux3 : Mux  Inputs=6
  Mux5 : Mux  Inputs=2
  Saturation1 : Saturate  UpperLimit=8.2  LowerLimit=0
  Sum of Elements : Sum  Inputs=+
  V_discrepancies : Sum  Inputs=+-
  V_was_there_a_discrepancy? : simulink/Logic and Bit Operations/Compare To Zero  relop=~=  OutDataTypeStr=boolean
  I1toI6 : Outport
  I_exceeded : Outport  Port=2
  wires:
  Mux5/1 -> I1toI6/1
  I/1 -> Gain4/1
  Gain4/1 -> V_discrepancies/2, Saturation1/1
  Mux2/1 -> Mux5/1
  Saturation1/1 -> V_discrepancies/1, Gain2/1
  Gain2/1 -> Demux1/1  "4"
  Mux3/1 -> Mux5/2
  Demux1/1 -> Mux2/1, Mux2/6
  Demux1/2 -> Mux2/2, Mux3/1
  Demux1/4 -> Mux2/3, Mux3/3
  Demux1/6 -> Mux2/4, Mux3/6
  Demux1/5 -> Mux2/5, Mux3/5
  Demux1/3 -> Mux3/2, Mux3/4
  V_discrepancies/1 -> Sum of Elements/1
  Sum of Elements/1 -> V_was_there_a_discrepancy?/1
  V_was_there_a_discrepancy?/1 -> I_exceeded/1

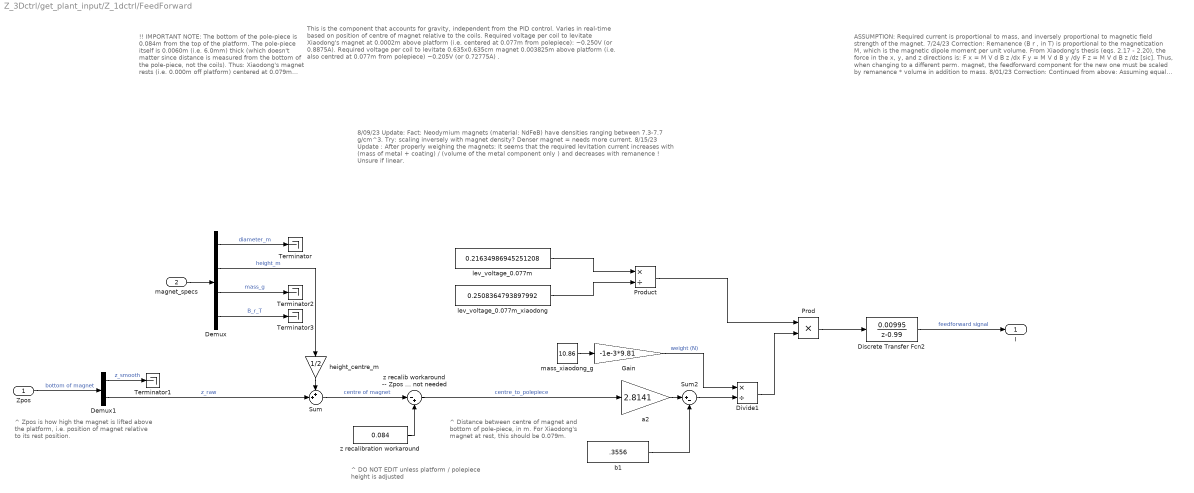
== system Z_3Dctrl/get_plant_input/Z_1dctrl/FeedForward ==
  note: ^ Zpos is how high the magnet is lifted above the platform, i.e. position of magnet relative to its rest position.
  note: 8/09/23 Update:
      |
      | Fact: Neodymium magnets (material: NdFeB) have densities ranging between 7.3-7.7 g/cm^3.
      | Try: scaling inversely with magnet density? Denser magnet = needs more current.
      |
      | 8/15/23 Update :
      | After properly weighing the magnets: It seems that the required levitation current increases with (mass of metal + coating) / (volume of the metal component only ) and decreases with remanence ! Unsure if linear.
  note: !! IMPORTANT NOTE:
      |
      | The bottom of the pole-piece is 0.084m from the top of the platform.
      | The pole-piece itself is 0.0060m (i.e. 6.0mm) thick (which doesn't matter since distance is measured from the bottom of the pole-piece, not the coils).
      |
      | Thus: Xiaodong's magnet rests (i.e. 0.000m off platform) centered at 0.079m from the polepiece (give or take 1mm due to deformity of the magnet).
  note: ASSUMPTION:
      | Required current is proportional to mass, and inversely proportional to magnetic field strength of the magnet.
      |
      | 7/24/23 Correction:
      | Remanence (B r , in T) is proportional to the magnetization M, which is the magnetic dipole moment per unit volume.
      |
      | From Xiaodong's thesis (eqs. 2.17 - 2.20), the force in the x, y, and z directions is:
      |
      | F x = M V d B z /dx
      |
      | F y = M V d B y /dy
      |
      | F z = M V d B z /dz [sic].
      |
      | Thus, when changing to a different perm. magnet, the feedforward component for the new one must be scaled by remanence * volume in addition to mass.
      |
      | 8/01/23 Correction:
      | Continued from above: Assuming equal density, volume scales with mass, and more volume = higher force produced but more mass = higher force required to levitate in the first place. Updated assumption: Any changes in mass will self-cancel due to corresponding changes in volume! (It's oversimplified and does not account for coating or the "b1" term to the left, but it's a step forward.)
  note: This is the component that accounts for gravity, independent from the PID control. Varies in real-time based on position of centre of magnet relative to the coils.
      |
      | Required voltage per coil to levitate Xiaodong's magnet at 0.0002m above platform (i.e. centered at 0.077m from polepiece): ~0.250V (or 0.8875A).
      |
      | Required voltage per coil to levitate 0.635x0.635cm magnet 0.003825m above platform (i.e. also centred at 0.077m from polepiece) ~0.205V (or 0.72775A) .
  note: ^ Distance between centre of magnet and bottom of pole-piece, in m.
      | For Xiaodong's magnet at rest, this should be 0.079m.
  note: ^ DO NOT EDIT unless platform / polepiece height is adjusted
  Zpos : Inport
  magnet_specs : Inport  Port=2
  Demux : Demux
  Demux1 : Demux  Outputs=2
  Discrete Transfer Fcn2 : DiscreteTransferFcn  Numerator=[0.00995]  Denominator=[1 -0.99]
  Divide1 : Product  Inputs=*/
  Gain : Gain  Gain=-1e-3*9.81
  Prod : Product  Inputs=**
  Product : Product  Inputs=*/
  Sum : Sum  Inputs=++|
  Sum2 : Sum  Inputs=|+-
  Terminator{,1..3} (4 alike) : Terminator
  a2 : Gain  Gain=2.8141
  b1 : Constant  Value=.3556
  height_centre_m : Gain  Gain=1/2
  lev_voltage_0.077m : Constant  Value=0.21634986945251208
  lev_voltage_0.077m_xiaodong : Constant  Value=0.2508364793897992
  mass_xiaodong_g : Constant  Value=10.86
  "z recalib workaround -- Zpos POSITIVE if not needed" : Sum  Inputs=|-+
  z recalibration workaround : Constant  Value=0.084
  I : Outport
  wires:
  a2/1 -> Sum2/1
  b1/1 -> Sum2/2
  Gain/1 -> Divide1/1  "weight (N)"
  Sum2/1 -> Divide1/2
  Divide1/1 -> Prod/2
  Prod/1 -> Discrete Transfer Fcn2/1
  "z recalib workaround -- Zpos POSITIVE if not needed"/1 -> a2/1  "centre_to_polepiece"
  z recalibration workaround/1 -> "z recalib workaround -- Zpos POSITIVE if not needed"/2
  Demux/1 -> Terminator/1  "diameter_m"
  magnet_specs/1 -> Demux/1
  Demux/3 -> Terminator2/1  "mass_g"
  Demux/4 -> Terminator3/1  "B_r_T"
  mass_xiaodong_g/1 -> Gain/1
  Demux/2 -> height_centre_m/1  "height_m"
  lev_voltage_0.077m/1 -> Product/1
  lev_voltage_0.077m_xiaodong/1 -> Product/2
  height_centre_m/1 -> Sum/1
  Sum/1 -> "z recalib workaround -- Zpos POSITIVE if not needed"/1  "centre of magnet"
  Product/1 -> Prod/1
  Zpos/1 -> Demux1/1  "bottom of magnet"
  Demux1/1 -> Terminator1/1  "z_smooth"
  Demux1/2 -> Sum/2  "z_raw"
  Discrete Transfer Fcn2/1 -> I/1  "feedforward signal"

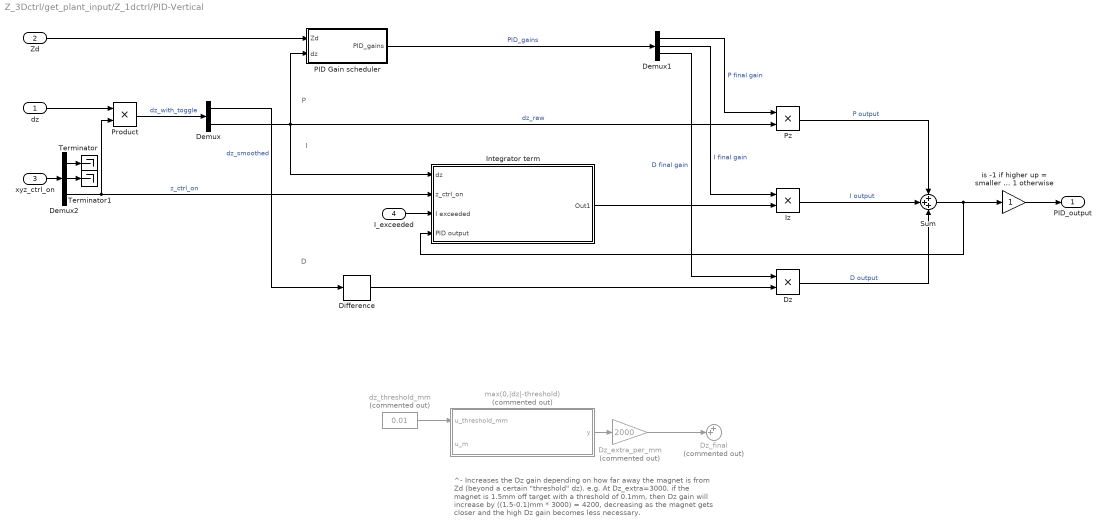
== system Z_3Dctrl/get_plant_input/Z_1dctrl/PID-Vertical ==
  note: P
  note: I
  note: D
  note: ^- Increases the Dz gain depending on how far away the magnet is from Zd (beyond a certain "threshold" dz).
      | e.g. At Dz_extra=3000, if the magnet is 1.5mm off target with a threshold of 0.1mm, then Dz gain will increase by ((1.5-0.1)mm * 3000) = 4200, decreasing as the magnet gets closer and the high Dz gain becomes less necessary.
  dz : Inport
  Zd : Inport  Port=2
  xyz_ctrl_on : Inport  Port=3
  I_exceeded : Inport  Port=4
  Demux : Demux  Outputs=2
  Demux1 : Demux  Outputs=3
  Demux2 : Demux  Outputs=3
  Difference : simulink/Discrete/Difference  ICPrevInput=0.0  OutMin=[]  OutMax=[]  OutDataType=fixdt(1, 16)  OutScaling=2^-10  DoSatur=off
  Dz : Product
  Dz_extra_per_mm : Gain  Commented=on  Gain=2000
  Dz_final : Sum  Commented=on  Inputs=++|
  Integrator term : Subsystem
  Iz : Product  Inputs=**
  PID Gain scheduler : Subsystem
  Product : Product
  Pz : Product  Inputs=**
  Sum : Sum  Inputs=+++
  Terminator : Terminator
  Terminator1 : Terminator
  dz_threshold_mm : Constant  Commented=on  Value=0.01
  "is -1 if higher up = smaller z, 1 otherwise" : Gain
  max(0,|dz|-threshold) : MATLAB Function  Commented=on  TreatAsAtomicUnit=on
  PID_output : Outport
  wires:
  Pz/1 -> Sum/1  "P output"
  Sum/1 -> "is -1 if higher up = smaller z, 1 otherwise"/1, Integrator term/4(PID output)
  "is -1 if higher up = smaller z, 1 otherwise"/1 -> PID_output/1
  Iz/1 -> Sum/2  "I output"
  Dz_extra_per_mm/1 -> Dz_final/2
  Dz/1 -> Sum/3  "D output"
  Difference/1 -> Dz/2
  max(0,|dz|-threshold)/1(y) -> Dz_extra_per_mm/1
  I_exceeded/1 -> Integrator term/3(I exceeded)
  Demux2/3 -> Product/2, Integrator term/2(z_ctrl_on)  "z_ctrl_on"
  Integrator term/1(Out1) -> Iz/2
  Demux/2 -> Integrator term/1(dz), PID Gain scheduler/2(dz), Pz/2  "dz_raw"
  dz/1 -> Product/1
  Demux/1 -> Difference/1  "dz_smoothed"
  Product/1 -> Demux/1  "dz_with_toggle"
  dz_threshold_mm/1 -> max(0,|dz|-threshold)/1(u_threshold_mm)
  PID Gain scheduler/1(PID_gains) -> Demux1/1  "PID_gains"
  Demux1/1 -> Pz/1  "P final gain"
  Demux1/2 -> Iz/1  "I final gain"
  Zd/1 -> PID Gain scheduler/1(Zd)
  Demux1/3 -> Dz/1  "D final gain"
  Demux2/1 -> Terminator/1
  Demux2/2 -> Terminator1/1
  xyz_ctrl_on/1 -> Demux2/1

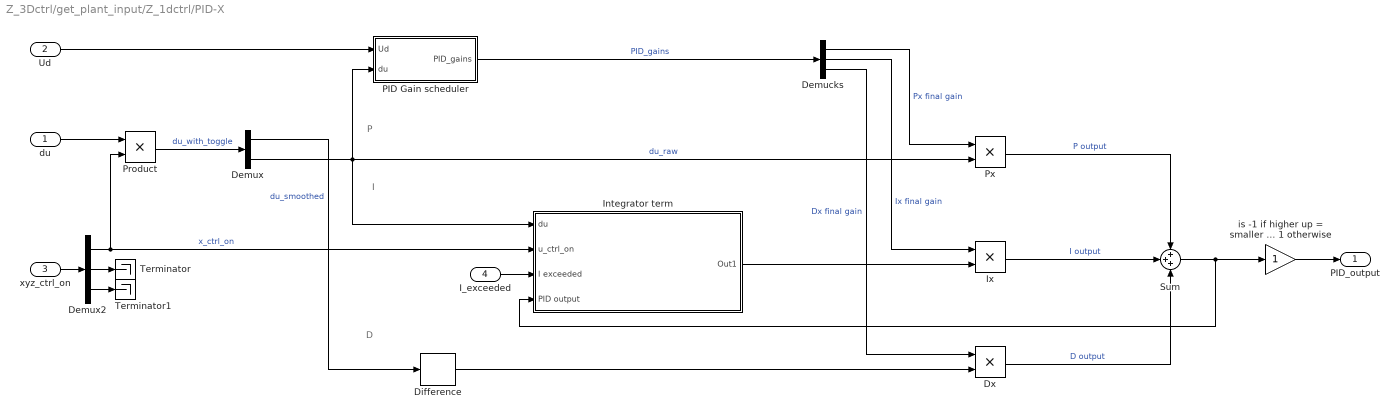
== system Z_3Dctrl/get_plant_input/Z_1dctrl/PID-X ==
  note: P
  note: I
  note: D
  du : Inport
  Ud : Inport  Port=2
  xyz_ctrl_on : Inport  Port=3
  I_exceeded : Inport  Port=4
  Demucks : Demux  Outputs=3
  Demux : Demux  Outputs=2
  Demux2 : Demux  Outputs=3
  Difference : simulink/Discrete/Difference  ICPrevInput=0.0  OutMin=[]  OutMax=[]  OutDataType=fixdt(1, 16)  OutScaling=2^-10  DoSatur=off
  Dx : Product
  Integrator term : Subsystem
  Ix : Product  Inputs=**
  PID Gain scheduler : Subsystem
  Product : Product
  Px : Product  Inputs=**
  Sum : Sum  Inputs=+++
  Terminator : Terminator
  Terminator1 : Terminator
  "is -1 if higher up = smaller z, 1 otherwise" : Gain
  PID_output : Outport
  wires:
  Px/1 -> Sum/1  "P output"
  Sum/1 -> "is -1 if higher up = smaller z, 1 otherwise"/1, Integrator term/4(PID output)
  "is -1 if higher up = smaller z, 1 otherwise"/1 -> PID_output/1
  Ix/1 -> Sum/2  "I output"
  Dx/1 -> Sum/3  "D output"
  Difference/1 -> Dx/2
  I_exceeded/1 -> Integrator term/3(I exceeded)
  Demux2/1 -> Integrator term/2(u_ctrl_on), Product/2  "x_ctrl_on"
  Integrator term/1(Out1) -> Ix/2
  Demux/2 -> Integrator term/1(du), PID Gain scheduler/2(du), Px/2  "du_raw"
  du/1 -> Product/1
  Demux/1 -> Difference/1  "du_smoothed"
  Product/1 -> Demux/1  "du_with_toggle"
  PID Gain scheduler/1(PID_gains) -> Demucks/1  "PID_gains"
  Demucks/1 -> Px/1  "Px final gain"
  Demucks/2 -> Ix/1  "Ix final gain"
  Ud/1 -> PID Gain scheduler/1(Ud)
  Demucks/3 -> Dx/1  "Dx final gain"
  Demux2/2 -> Terminator/1
  Demux2/3 -> Terminator1/1
  xyz_ctrl_on/1 -> Demux2/1

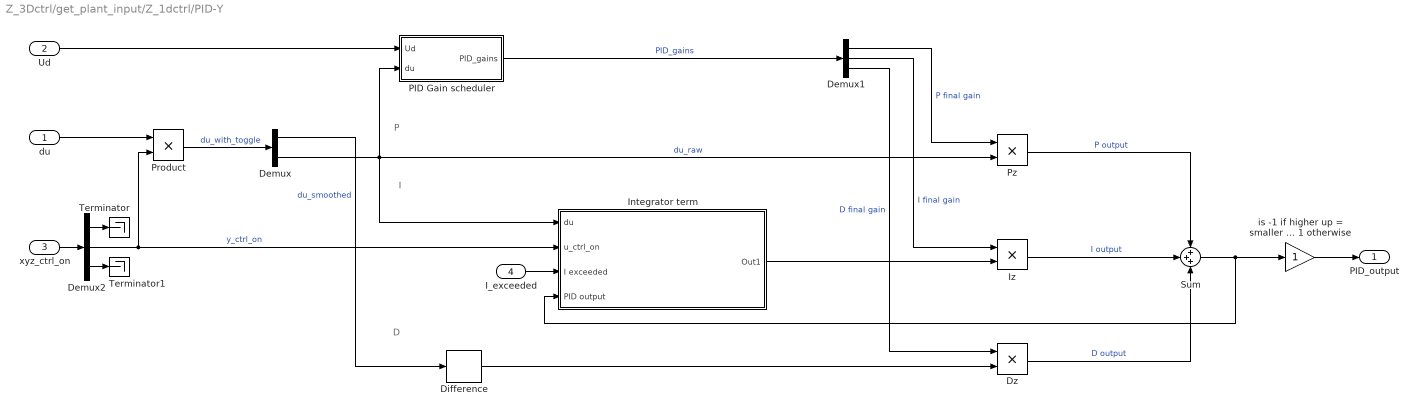
== system Z_3Dctrl/get_plant_input/Z_1dctrl/PID-Y ==
  note: P
  note: I
  note: D
  du : Inport
  Ud : Inport  Port=2
  xyz_ctrl_on : Inport  Port=3
  I_exceeded : Inport  Port=4
  Demux : Demux  Outputs=2
  Demux1 : Demux  Outputs=3
  Demux2 : Demux  Outputs=3
  Difference : simulink/Discrete/Difference  ICPrevInput=0.0  OutMin=[]  OutMax=[]  OutDataType=fixdt(1, 16)  OutScaling=2^-10  DoSatur=off
  Dz : Product
  Integrator term : Subsystem
  Iz : Product  Inputs=**
  PID Gain scheduler : Subsystem
  Product : Product
  Pz : Product  Inputs=**
  Sum : Sum  Inputs=+++
  Terminator : Terminator
  Terminator1 : Terminator
  "is -1 if higher up = smaller z, 1 otherwise" : Gain
  PID_output : Outport
  wires:
  Pz/1 -> Sum/1  "P output"
  Sum/1 -> "is -1 if higher up = smaller z, 1 otherwise"/1, Integrator term/4(PID output)
  "is -1 if higher up = smaller z, 1 otherwise"/1 -> PID_output/1
  Iz/1 -> Sum/2  "I output"
  Dz/1 -> Sum/3  "D output"
  Difference/1 -> Dz/2
  I_exceeded/1 -> Integrator term/3(I exceeded)
  Demux2/2 -> Product/2, Integrator term/2(u_ctrl_on)  "y_ctrl_on"
  Integrator term/1(Out1) -> Iz/2
  Demux/2 -> Integrator term/1(du), PID Gain scheduler/2(du), Pz/2  "du_raw"
  du/1 -> Product/1
  Demux/1 -> Difference/1  "du_smoothed"
  Product/1 -> Demux/1  "du_with_toggle"
  PID Gain scheduler/1(PID_gains) -> Demux1/1  "PID_gains"
  Demux1/1 -> Pz/1  "P final gain"
  Demux1/2 -> Iz/1  "I final gain"
  Ud/1 -> PID Gain scheduler/1(Ud)
  Demux1/3 -> Dz/1  "D final gain"
  Demux2/1 -> Terminator/1
  Demux2/3 -> Terminator1/1
  xyz_ctrl_on/1 -> Demux2/1

== system Z_3Dctrl/get_plant_input/Z_1dctrl/Wrench scheduling ==
  XYZ_SAR : Inport
  PID_YXZ[3x1] : Inport  Port=2
  CAM[6x3]_BASE : Constant  Value=|
      | [    0.6670    0.3916    0.1667
      |     0.0748    0.6938    0.1667
      |    -0.6052    0.4567    0.1667
      |    -0.6327   -0.3547    0.1667
      |     0.0652   -0.8502    0.1667
      |     0.7651   -0.5238    0.1667]
  CAM[6x3]_CHUNK01 : Constant  Value=|
      | [    1.3910    0.3620    0.1667
      |     0.4079    0.7676    0.1667
      |    -1.8144    1.2338    0.1667
      |    -1.9457   -0.6900    0.1667
      |     0.6358   -0.6984    0.1667
      |     1.1892   -0.2089    0.1667]
  CAM[6x3]_CHUNK02 : Constant  Value=|
      | [    1.3581    0.4248    0.1667
      |     0.4244    1.0097    0.1667
      |    -1.7217    0.8668    0.1667
      |    -1.8700   -0.7631    0.1667
      |     0.6047   -1.0153    0.1667
      |     1.1354   -0.3480    0.1667]
  CAM[6x3]_xiaodong : Constant  Commented=on  Value=|
      | [0.2500    0.0833    0.1667
      |          0    0.1667    0.1667
      |    -0.2500    0.0833    0.1667
      |    -0.2500   -0.0833    0.1667
      |          0   -0.1667    0.1667
      |     0.2500   -0.0833    0.1667]
  Demux : Demux  Outputs=3
  basic_mode : Constant  Value=0
  box_base_XYcols : Constant  Value=|
      | [-2.5, -2.7,
      | 2.0, 2.3]
  box_chunk01_XYcols : Constant  Value=|
      | [-3.32, 1.8,
      | 5.02, 12.889]
  box_chunk02_XYcols : Constant  Value=|
      | [-3.32, -10.47,
      | 5.02, -1.7]
  wrench_scheduler : MATLAB Function  TreatAsAtomicUnit=on
  PID_out : Outport
  wires:
  PID_YXZ[3x1]/1 -> wrench_scheduler/4(PID_XYZ)
  wrench_scheduler/1(PID_out) -> PID_out/1
  CAM[6x3]_BASE/1 -> wrench_scheduler/5(wrench_base)
  CAM[6x3]_CHUNK01/1 -> wrench_scheduler/6(wrench_chunk01)
  CAM[6x3]_CHUNK02/1 -> wrench_scheduler/7(wrench_chunk02)
  box_base_XYcols/1 -> wrench_scheduler/8(box_base)
  box_chunk01_XYcols/1 -> wrench_scheduler/9(box_chunk01)
  box_chunk02_XYcols/1 -> wrench_scheduler/10(box_chunk02)
  XYZ_SAR/1 -> Demux/1
  Demux/1 -> wrench_scheduler/1(X_SAR)  "x_SAR"
  Demux/2 -> wrench_scheduler/2(Y_SAR)  "y_SAR"
  Demux/3 -> wrench_scheduler/3(Z_SAR)  "z_SAR"
  basic_mode/1 -> wrench_scheduler/11(basic_mode)
